simulink model "nonlinear_model"  (R2018a)
settings: Solver=ode45  StartTime=0.0  StopTime=10.0  RelTol=1e-3  EnableMultiTasking=on
values from neighbouring files (symbols this model uses):
  g = 9.81    [gibalo_system_model.m]
  J_bz = 8922223.33e-9 + m_b*l^2    (= 0.0139543664174)    [gibalo_system_model.m]
  l = 0.06721    [gibalo_system_model.m]
  m_b = 1.114    [gibalo_system_model.m]
settings Model: Creator=antun  LastModifiedBy=Gospar
settings DataIOCC: LimitDataPoints=on  SaveFormat=Array
settings OptimizationCC: LifeSpan=inf
settings DebuggingCC: SFUnexpectedBacktrackingDiag=warning  SFNoUnconditionalDefaultTransitionDiag=warning  SFExecutionAtInitializationDiag=none
settings HardwareCC: ProdBitPerPointer=32  ProdBitPerSizeT=32  ProdBitPerPtrDiffT=32  ProdLargestAtomicFloat=None  ProdIntDivRoundTo=Undefined  ProdEndianess=Unspecified  ProdWordSize=32  ProdHWDeviceType=32-bit Generic
settings ModelReferenceCC: PropagateSignalLabelsOutOfModel=off
settings CodeAppCC: StateflowObjectComments=on
settings GRTTargetCC: TargetLangStandard=C89/C90 (ANSI)  GeneratePreprocessorConditionals=Disable all
settings ConfigComp: CovMetricSettings=dw  CovHtmlReporting=on  CovSaveCumulativeToWorkspaceVar=on  CovSaveSingleToWorkspaceVar=on  CovExternalEMLEnable=off

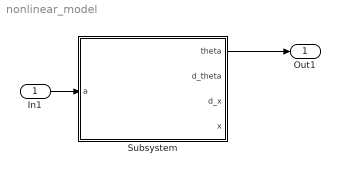
== system nonlinear_model ==
  In1 : Inport
  Subsystem : Subsystem
  Out1 : Outport
  wires:
  In1/1 -> Subsystem/1(a)
  Subsystem/1(theta) -> Out1/1

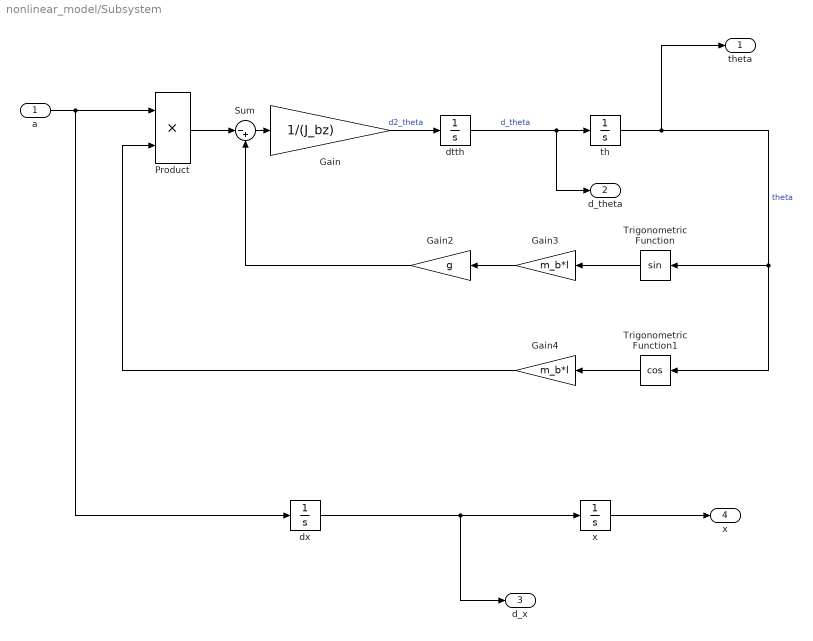
== system nonlinear_model/Subsystem ==
  a : Inport
  Gain : Gain  Gain=1/(J_bz)
  Gain2 : Gain  Gain=g
  Gain3 : Gain  Gain=m_b*l
  Gain4 : Gain  Gain=m_b*l
  Product : Product
  Sum : Sum  Inputs=|-+
  Trigonometric Function : Trigonometry
  Trigonometric Function1 : Trigonometry  Operator=cos
  dtth : Integrator
  dx : Integrator
  th : Integrator
  "x   " : Integrator
  theta : Outport
  d_theta : Outport  Port=2
  d_x : Outport  Port=3
  x : Outport  Port=4
  wires:
  Gain/1 -> dtth/1  "d2_theta"
  Product/1 -> Sum/1
  Gain2/1 -> Sum/2
  th/1 -> theta/1, Trigonometric Function/1, Trigonometric Function1/1  "theta"
  dtth/1 -> d_theta/1, th/1  "d_theta"
  Sum/1 -> Gain/1
  Trigonometric Function/1 -> Gain3/1
  dx/1 -> d_x/1, "x   "/1
  a/1 -> dx/1, Product/1
  "x   "/1 -> x/1
  Trigonometric Function1/1 -> Gain4/1
  Gain3/1 -> Gain2/1
  Gain4/1 -> Product/2
